simulink model "MPC_KF"  (R2022a)
settings: Solver=VariableStepAuto  StartTime=0.0  StopTime=20  RelTol=1e-3
values from neighbouring files (symbols this model uses):
  B_noise = [sysd.B ones(size(sysd.B,1),1)]    [main.m]
  C_states = eye(length(A))    [main.m]
  D_noise = [D_states zeros(size(D_states,1),1)]    [main.m]
  N5 = 100    [main.m]
  NK = zeros(4,3)    [main.m]
  Q5 = Q_d    [main.m]
  R5 = R_d    (= 10000)    [main.m]
  RK = 10*blkdiag(1,1,1)    [main.m]
  S5 = P_d    [main.m]
  sysd = c2d(sys,T_sampling)    [main.m]
  Ts = T_sampling    [main.m]
  u_max = deg2rad(15)    [main.m]
  u_min = deg2rad(-15)    [main.m]
  x0 = [deg2rad(0) deg2rad(15) 0 -300]    [main.m]
  x_ref = [0 0 0 0]    [main.m]
undefined symbols (not defined in the file or in its folder): Discrete, mpc_point_3, Time
libraries: simulink x2, ctrlSharedLib x1
settings Model: LastModifiedBy=david
settings OptimizationCC: BlockReduction=off  BooleanDataType=off
settings DebuggingCC: SaveWithParameterizedLinksMsg=none  UnderspecifiedInitializationDetection=Classic  MergeDetectMultiDrivingBlocksExec=none  SignalResolutionControl=TryResolveAllWithWarning
settings HardwareCC: TargetUnknown=on
settings ModelReferenceCC: PropagateSignalLabelsOutOfModel=off

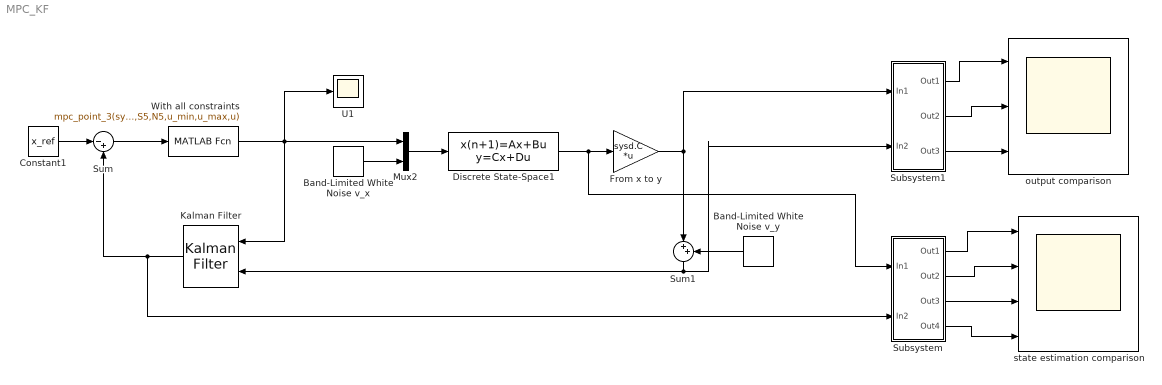
== system MPC_KF ==
  "Band-Limited White Noise v_x " : simulink/Sources/Band-Limited White Noise  Cov=power_vx  Ts=Ts  seed=[23341]
  Band-Limited White Noise v_y : simulink/Sources/Band-Limited White Noise  Cov=power_vy  Ts=Ts  seed=[1258]
  Constant1 : Constant  Value=x_ref
  Discrete State-Space1 : DiscreteStateSpace  A=sysd.A  B=B_noise  C=C_states  D=D_noise  InitialCondition=x0  SampleTime=Ts
  From x to y : Gain  Gain=sysd.C  Multiplication=Matrix(K*u)
  Kalman Filter : ctrlSharedLib/Kalman Filter  TimeDomain=Discrete-Time  UseCurrentEstimator=off  ModelSource=Individual A, B, C, D matrices  ModelSourceVariable=ss(0.95,1,1,0,1)  A=sysd.A  B=sysd.B  C=sysd.C  D=sysd.D  NumberOfStates=1  NumberOfInputs=1  NumberOfOutputs=1  InitialEstimateSource=Dialog  X0=x0  P0=10  UseK=off  UseGH=off  NumberOfProcessNoiseInputs=1  G=1  TimeInvariantG=on  H=0  TimeInvariantH=on  Q=QK  TimeInvariantQ=on  R=RK  TimeInvariantR=on  N=NK  TimeInvariantN=on  AddInputPort=on  AddEnablePort=off  OutputEstimatedY=off  OutputP=off  Ts=Ts
  Mux2 : Mux  Inputs=2
  Subsystem : Subsystem
  Subsystem1 : Subsystem
  Sum : Sum  Inputs=|-+
  Sum1 : Sum  Inputs=|++
  U1 : Scope
  With all constraints : MATLABFcn  MATLABFcn=mpc_point_3(sysd.A,sysd.B,Q5,R5,S5,N5,u_min,u_max,u)  OutputDimensions=1
  output comparison : Scope  NumInputPorts=3
  "state estimation comparison " : Scope  NumInputPorts=4
  wires:
  Sum/1 -> With all constraints/1
  From x to y/1 -> Subsystem1/1(In1), Sum1/1
  With all constraints/1 -> Kalman Filter/1, Mux2/1, U1/1
  Constant1/1 -> Sum/1
  "Band-Limited White Noise v_x "/1 -> Mux2/2
  Band-Limited White Noise v_y/1 -> Sum1/2
  Sum1/1 -> Subsystem1/2(In2), Kalman Filter/2
  Kalman Filter/1 -> Subsystem/2(In2), Sum/2
  Discrete State-Space1/1 -> Subsystem/1(In1), From x to y/1
  Mux2/1 -> Discrete State-Space1/1
  Subsystem/1(Out1) -> "state estimation comparison "/1
  Subsystem/2(Out2) -> "state estimation comparison "/2
  Subsystem/3(Out3) -> "state estimation comparison "/3
  Subsystem/4(Out4) -> "state estimation comparison "/4
  Subsystem1/1(Out1) -> output comparison/1
  Subsystem1/2(Out2) -> output comparison/2
  Subsystem1/3(Out3) -> output comparison/3

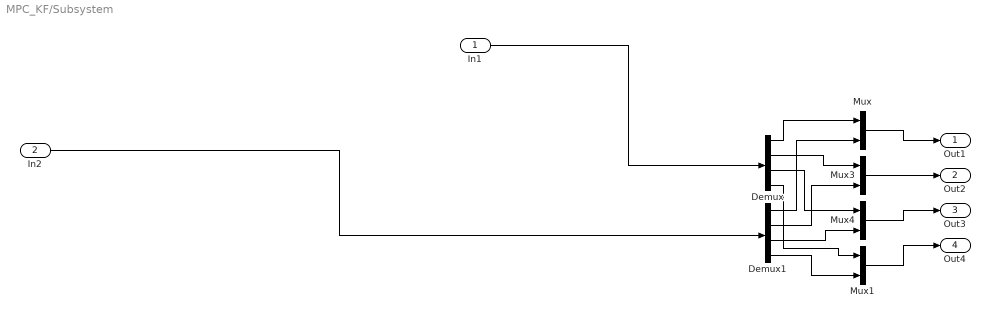
== system MPC_KF/Subsystem ==
  In1 : Inport
  In2 : Inport  Port=2
  Demux : Demux
  Demux1 : Demux
  Mux{,1,3..4} (4 alike) : Mux  Inputs=2
  Out1 : Outport
  Out2 : Outport  Port=2
  Out3 : Outport  Port=3
  Out4 : Outport  Port=4
  wires:
  Demux/1 -> Mux/1
  Demux1/4 -> Mux1/2
  Demux1/1 -> Mux/2
  Demux1/3 -> Mux4/2
  Demux/3 -> Mux4/1
  Demux1/2 -> Mux3/2
  Mux1/1 -> Out4/1
  Demux/4 -> Mux1/1
  Demux/2 -> Mux3/1
  In2/1 -> Demux1/1
  Mux/1 -> Out1/1
  Mux3/1 -> Out2/1
  Mux4/1 -> Out3/1
  In1/1 -> Demux/1

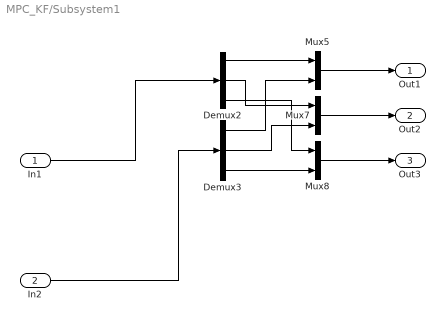
== system MPC_KF/Subsystem1 ==
  In1 : Inport
  In2 : Inport  Port=2
  Demux2 : Demux  Outputs=3
  Demux3 : Demux  Outputs=3
  Mux5 : Mux  Inputs=2
  Mux7 : Mux  Inputs=2
  Mux8 : Mux  Inputs=2
  Out1 : Outport
  Out2 : Outport  Port=2
  Out3 : Outport  Port=3
  wires:
  Demux2/1 -> Mux5/1
  Demux3/2 -> Mux7/2
  Demux2/2 -> Mux7/1
  Demux3/1 -> Mux5/2
  Demux2/3 -> Mux8/1
  Demux3/3 -> Mux8/2
  In1/1 -> Demux2/1
  Mux8/1 -> Out3/1
  In2/1 -> Demux3/1
  Mux7/1 -> Out2/1
  Mux5/1 -> Out1/1
